simulink model "ExampleHovercraft"  (Simulink 9.2)
settings: Solver=FixedStepDiscrete  StartTime=0.0  StopTime=inf  FixedStep=0.001  RelTol=1e-3  EnableMultiTasking=on
libraries: rFproPhysicsLib x6
settings Model: Creator=enewton  LastModifiedBy=SeanKavanagh  TunableVars=LOCAL_PORT_RECV,REMOTE_PORT_RECV  TunableVarsStorageClass=Auto,Auto  TunableVarsTypeQualifier=,
settings DataIOCC: SaveOutput=off  SignalLogging=off  DSMLogging=off  SaveTime=off
settings OptimizationCC: DefaultParameterBehavior=Inlined  ExpressionDepthLimit=2147483647
settings DebuggingCC: SolverPrmCheckMsg=warning
settings HardwareCC: TargetBitPerPointer=64  TargetBitPerSizeT=64  TargetBitPerPtrDiffT=64  TargetLongLongMode=on  TargetIntDivRoundTo=Zero  TargetEndianess=LittleEndian  TargetWordSize=64  TargetHWDeviceType=MATLAB Host  ProdEqTarget=off
settings RTWCC: SystemTargetFile=rfpro.tlc  MakeCommand="make_rtw OPTS=\"-DRUN_PHYSICS\""  TemplateMakefile=rfpro.tmf  Description=rFpro Target (Run Physics)  TargetLang=C++
settings STFCustomTargetCC: ModelReferenceCompliant=off  GeneratePreprocessorConditionals=Disable all  CombineOutputUpdateFcns=on  MatFileLogging=on  CPPClassGenCompliant=on  GRTInterface=off  SystemTargetFile=rfpro.tlc
settings GRTTargetCC: ModelReferenceCompliant=off  ParMdlRefBuildCompliant=off  CompOptLevelCompliant=off  ConcurrentExecutionCompliant=off  CombineOutputUpdateFcns=on  GRTInterface=off  UseToolchainInfoCompliant=off

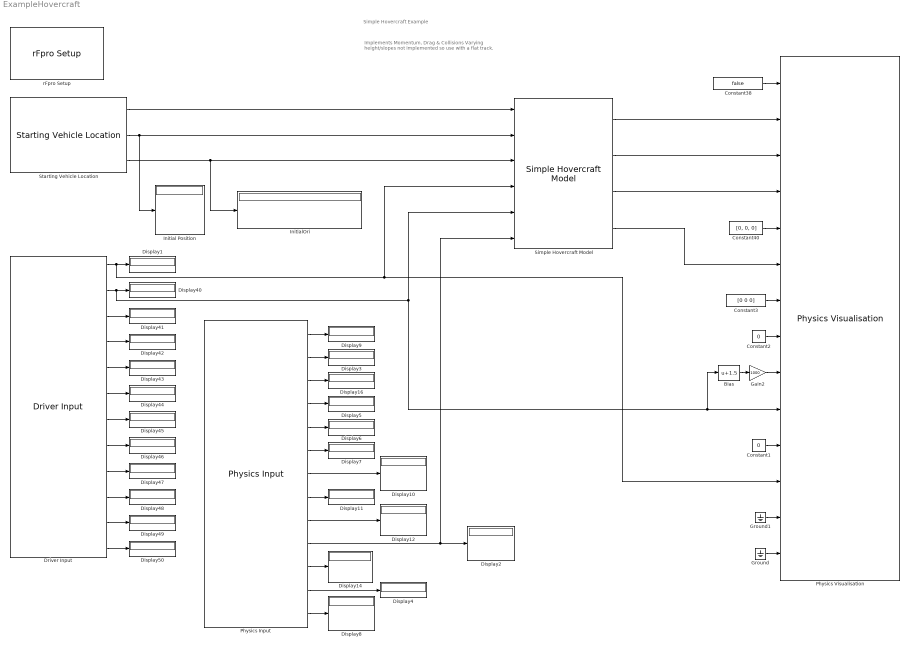
== system ExampleHovercraft ==
  note: Simple Hovercraft Example
  note: Implements Momentum, Drag & Collisions
      | Varying height/slopes not implemented
      | so use with a flat track.
  Bias : Bias  Bias=1.5
  Constant1 : Constant  Value=0  OutDataTypeStr=double
  Constant2 : Constant  Value=0  OutDataTypeStr=int32
  Constant3 : Constant  Value=[0 0 0]  OutDataTypeStr=double
  Constant38 : Constant  Value=false
  Constant40 : Constant  Value=[0, 0, 0]
  Display{1..12,14,16,40..50} (25 alike) : Display
  Driver Input : rFproPhysicsLib/Driver Input
  Gain2 : Gain  Gain=1000
  Ground : Ground
  Ground1 : Ground
  Initial Position : Display
  InitialOri : Display
  Physics Input : rFproPhysicsLib/Physics Input
  Physics Visualisation : rFproPhysicsLib/Physics Visualisation  PAR_SKIP_INTERNAL_PHYSICS=off  PAR_ACCEL_VALID=on  PAR_ROT_ACCEL_VALID=off  PAR_GEAR_VALID=off  PAR_RPM_VALID=on  PAR_INPUTS_VALID=on  PAR_STEER_TORQUE_VALID=off  PAR_HEADLIGHTS_ON_VALID=off  PAR_WHEEL_POS_VALID=off  PAR_WHEEL_ORI_VALID=off  PAR_TYRE_PARAMS_VALID=off  PAR_WHEEL_ROTATION_VALID=off  PAR_WHEEL_BRAKE_TEMP_VALID=off  PAR_WHEEL_TREAD_TEMP_VALID=off  PAR_WHEEL_AIR_TEMP_VALID=off  period=-1  offset=0  useReverseByteOrder=on  rFpro__platform=Remote Model - Default
  Simple Hovercraft Model : rFproPhysicsLib/Internal Utility/Simple Hovercraft Model  MASS=600  C_DRAG=0.7  TIMESTEP=0.001
  Starting Vehicle Location : rFproPhysicsLib/Starting Vehicle Location  cg_offset=[-2, 0, 0.575]  numPackets=2  rFpro__platform=Remote Model - Default
  rFpro Setup : rFproPhysicsLib/rFpro Setup  platform=Remote Model - Default  stopOnSessionEnd=on  usePseudoRealtime=on  syncToRF=on  useReverseByteOrder=off  useRfTime=on  minIterations=4  maxIterations=1000  ipReceiveAddress='127.0.0.1'  ipReceivePort=11054  receiveSampleTime=-1  ipTransmitAddress='127.0.0.1'  ipTransmitPort=11052  transmitSampleTime=-1  pluginType=RUN_PHYSICS  sysTarget=xpctarget.tlc  templateMakeFile=xpc_default_tmf  makeCommand=make_rtw  buildDesc=xPC target
  wires:
  Constant38/1 -> Physics Visualisation/1
  Constant40/1 -> Physics Visualisation/5
  Constant1/1 -> Physics Visualisation/11
  Physics Input/2 -> Display3/1
  Physics Input/3 -> Display16/1
  Physics Input/4 -> Display5/1
  Physics Input/5 -> Display6/1
  Physics Input/6 -> Display7/1
  Physics Input/10 -> Simple Hovercraft Model/6, Display2/1
  Physics Input/11 -> Display14/1
  Driver Input/3 -> Display41/1
  Driver Input/4 -> Display42/1
  Driver Input/5 -> Display43/1
  Driver Input/6 -> Display44/1
  Driver Input/7 -> Display45/1
  Driver Input/8 -> Display46/1
  Driver Input/9 -> Display47/1
  Driver Input/10 -> Display48/1
  Driver Input/11 -> Display49/1
  Driver Input/12 -> Display50/1
  Constant3/1 -> Physics Visualisation/7
  Gain2/1 -> Physics Visualisation/9
  Driver Input/1 -> Simple Hovercraft Model/4, Physics Visualisation/12, Display1/1
  Starting Vehicle Location/3 -> Simple Hovercraft Model/3, InitialOri/1
  Starting Vehicle Location/2 -> Simple Hovercraft Model/2, Initial Position/1
  Simple Hovercraft Model/3 -> Physics Visualisation/4
  Simple Hovercraft Model/1 -> Physics Visualisation/2
  Simple Hovercraft Model/4 -> Physics Visualisation/6
  Simple Hovercraft Model/2 -> Physics Visualisation/3
  Driver Input/2 -> Simple Hovercraft Model/5, Bias/1, Physics Visualisation/10, Display40/1
  Ground1/1 -> Physics Visualisation/13
  Physics Input/9 -> Display12/1
  Physics Input/7 -> Display10/1
  Physics Input/12 -> Display4/1
  Physics Input/13 -> Display8/1
  Physics Input/1 -> Display9/1
  Ground/1 -> Physics Visualisation/14
  Constant2/1 -> Physics Visualisation/8
  Starting Vehicle Location/1 -> Simple Hovercraft Model/1
  Physics Input/8 -> Display11/1
  Bias/1 -> Gain2/1
